simulink model "GPC_model"  (R2022b)
settings: Solver=FixedStepAuto  StartTime=0.0  StopTime=100  FixedStep=0.1  RelTol=1e-3  AbsTol=1e-6
undefined symbols (not defined in the file): DiscIntNeverNeededParam, Ks, Ts
settings Model: ExtModeTrigDuration=12000  ExtModeTrigLevel=0.400000  Creator=jims  LastModifiedBy=artur
settings SolverCC: AutoScaleAbsTol=off  AlgebraicLoopSolver=TrustRegion
settings DataIOCC: ExternalInput=[]  InitialState=[]  MaxDataPoints=5000  SaveFormat=Array  SignalLoggingSaveFormat=ModelDataLogs  SaveOutput=off  SaveTime=off  ReturnWorkspaceOutputs=off  SignalLoggingName=sigsOut
settings OptimizationCC: BooleanDataType=off  ExpressionDepthLimit=2147483647  LifeSpan=inf
settings DebuggingCC: SaveWithParameterizedLinksMsg=none  UnderspecifiedInitializationDetection=Classic  MergeDetectMultiDrivingBlocksExec=none  SignalResolutionControl=TryResolveAllWithWarning  MultiTaskDSMMsg=warning  MultiTaskCondExecSysMsg=none  IntegerOverflowMsg=none  FcnCallInpInsideContextMsg=warning  UnconnectedInputMsg=warning  UnconnectedOutputMsg=warning  UnconnectedLineMsg=warning  AllowSymbolicDim=off  StateNameClashWarn=warning  PregeneratedLibrarySubsystemCodeDiagnostic=none  SFUnexpectedBacktrackingDiag=warning  SFNoUnconditionalDefaultTransitionDiag=warning  SFExecutionAtInitializationDiag=none  SFMachineParentedDataDiag=warning  IntegerSaturationMsg=none  ArithmeticOperatorsInVariantConditions=warning
settings HardwareCC: ProdBitPerLong=64  ProdHWDeviceType=Intel->x86-64 (Linux 64)  TargetBitPerLong=64  TargetBitPerPointer=64  TargetIntDivRoundTo=Zero  TargetEndianess=LittleEndian  TargetWordSize=64  TargetHWDeviceType=Intel->x86-64
settings ModelReferenceCC: EnableRefExpFcnMdlSchedulingChecks=on  PropagateSignalLabelsOutOfModel=off
settings SFSimCC: SimUseLocalCustomCode=off  CustomCodeUndefinedFunction=UseInterfaceOnly
settings RTWCC: Description=Simulink Desktop Real-Time  SystemTargetFile=sldrt.tlc  TemplateMakefile=sldrt.tmf  RTWUseLocalCustomCode=off  RTWCompilerOptimization=on
settings CodeAppCC: MaxIdLength=95  StateflowObjectComments=on
settings SimulinkDesktopRealTimeCC: TargetLibSuffix=_sldrt.a  TargetPreCompLibLocation=C:\Program Files\MATLAB\R2022b\toolbox\sldrt\lib\win64  TargetLangStandard=C89/C90 (ANSI)  SupportVariableSizeSignals=off
settings ConfigComp: CovMetricSettings=dw  CovSaveCumulativeToWorkspaceVar=on  CovSaveSingleToWorkspaceVar=on  CovExternalEMLEnable=off

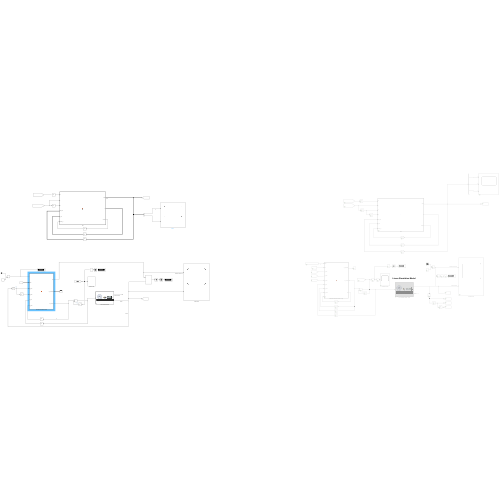
[thumbnail: Simulink's stored preview of the top-level diagram]
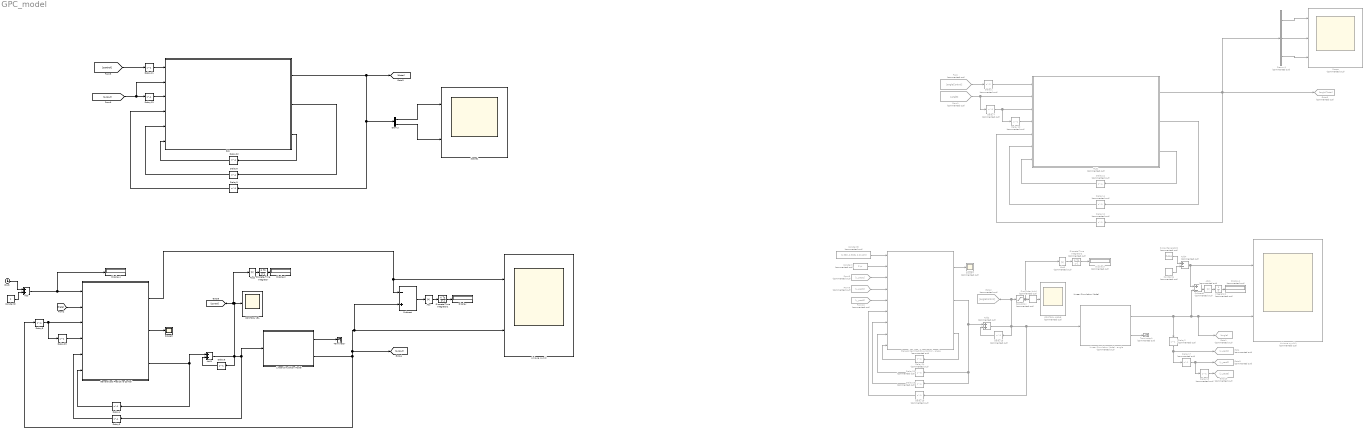
== system GPC_model ==
  note: Linear Simulation Model
  Abs : Abs  SaturateOnIntegerOverflow=off
  Abs1 : Abs  Commented=on  SaturateOnIntegerOverflow=off
  Abs2 : Abs  SaturateOnIntegerOverflow=off
  Abs3 : Abs  Commented=on  SaturateOnIntegerOverflow=off
  Add : Sum
  Add1 : Sum
  Add2 : Sum  Commented=on
  Add4 : Sum  Commented=on  Inputs=+-
  CONTROL ANGLE : Scope  Commented=on
  CONTROL VEL : Scope
  Clock : Clock
  Constant : Constant  Commented=on  Value=2*pi
  Constant2 : Constant
  Constant3 : Constant  Commented=on  Value=[1.988 -0.9884 0.01129]
  Constant4 : Constant  Commented=on  Value=2*3.14
  Delay1 : Delay  Commented=on  InitialCondition=0
  Delay{2,7,10,15..19} (8 alike) : Delay  Commented=on  DelayLength=1  InitialCondition=0
  Delay{3..6,11,13,23} (7 alike) : Delay  DelayLength=1  InitialCondition=0
  Delay12 : Delay  Commented=on  DelayLength=1  InitialCondition=[2.05 -0.95 0.01]
  Delay14 : Delay  Commented=on  DelayLength=1  InitialCondition=eye(3) * 10^6
  Delay20 : Delay  Commented=on  InitialCondition=0
  Delay21 : Delay  Commented=on  DelayLength=1  InitialCondition=10
  Delay22 : Delay  DelayLength=1  InitialCondition=10
  Delay24 : Delay  Commented=on  DelayLength=1  InitialCondition=1
  Delay8 : Delay  DelayLength=1  InitialCondition=eye(2) * 10^6
  Delay9 : Delay  DelayLength=1  InitialCondition=[0.85 21]
  Demux : Demux  Outputs=2
  Demux1 : Demux  Commented=on  Outputs=3
  Discrete-Time Integrator : DiscreteIntegrator  SampleTime=-1  ICPrevOutput=DiscIntNeverNeededParam  ICPrevScaledInput=DiscIntNeverNeededParam
  Discrete-Time Integrator1 : DiscreteIntegrator  SampleTime=-1  ICPrevOutput=DiscIntNeverNeededParam  ICPrevScaledInput=DiscIntNeverNeededParam
  Discrete-Time Integrator2 : DiscreteIntegrator  Commented=on  SampleTime=-1  ICPrevOutput=DiscIntNeverNeededParam  ICPrevScaledInput=DiscIntNeverNeededParam
  Display : Display
  Display1 : Display  Commented=on
  Display2 : Display
  Display3 : Display  Commented=on
  Display4 : Display
  First Order Hold : FirstOrderHold  Commented=on  ErrorTolerance=inf
  From : From  Commented=on  GotoTag=angleControl
  From1 : From  Commented=on  GotoTag=angle
  From10 : From  Commented=on  GotoTag=y_past3
  From8 : From  Commented=on  GotoTag=y_past1
  From9 : From  Commented=on  GotoTag=y_past2
  Generalized Predictive Control : MATLAB Function  TreatAsAtomicUnit=on
  Generalized Predictive Control - angle : MATLAB Function  Commented=on  TreatAsAtomicUnit=on
  Goto : Goto  Commented=on  GotoTag=y_past1
  Goto1 : Goto  Commented=on  GotoTag=angle
  Goto10 : Goto  Commented=on  GotoTag=y_past3
  Goto2 : Goto  Commented=on  GotoTag=angleControl
  Goto5 : Goto  Commented=on  GotoTag=angleTheta
  Goto9 : Goto  Commented=on  GotoTag=y_past2
  Integrator1 : Integrator  Commented=on
  Linear Simulation Model : Subsystem  mask{x0=[0*25*pi/2 0]}
      mask prompts: x0 "Initial conditions [angle vel]"
      mask Display: image(imread('Servo_m.JPG'))
  Linear Simulation Model - angle : Subsystem  Commented=on  mask{x0=[0 0]}
      mask prompts: x0 "Initial conditions [angle vel]"
      mask Display: image(imread('Servo_m.JPG'))
  Liniowe wyniki : Scope  NumInputPorts=2
  Liniowe wyniki1 : Scope  Commented=on  NumInputPorts=2
  Pulse Generator2 : DiscretePulseGenerator  Commented=on  PulseType=Time based  Amplitude=4*pi  Period=4  PulseWidth=50
  RLS : MATLAB Function  TreatAsAtomicUnit=on
  RLS1 : MATLAB Function  Commented=on  TreatAsAtomicUnit=on
  Saturation : Saturate  Commented=on  UpperLimit=1  LowerLimit=-1
  Scope : Scope  Commented=on  NumInputPorts=3
  Scope1 : Scope  NumInputPorts=2
  Scope3 : Scope
  Scope4 : Scope  Commented=on
  Subtract : Sum  Inputs=-+
  Subtract1 : Sum  Commented=on  Inputs=+-
  Terminator : Terminator
  Terminator1 : Terminator  Commented=on
  wires:
  Demux/2 -> Scope1/2  "b1"
  Generalized Predictive Control/3(du_control) -> Add1/1, Delay4/1  "du"
  Delay11/1 -> RLS/1(u1)
  Demux/1 -> Scope1/1  "a1"
  Delay9/1 -> RLS/4(theta_old)
  [control] -> Delay11/1
  Delay4/1 -> Generalized Predictive Control/6(du_past)
  RLS/1(theta) -> Demux/1, Delay9/1, [theta]  "theta"
  Generalized Predictive Control/2(du_predicted) -> Scope3/1
  Delay13/1 -> RLS/3(y1)
  [output] -> Delay13/1, RLS/2(y)
  RLS/2(P) -> Delay8/1
  Delay8/1 -> RLS/5(P_old)
  Delay3/1 -> Generalized Predictive Control/5(u_past)
  [theta] -> Generalized Predictive Control/2(theta)
  Delay6/1 -> Add1/2
  Generalized Predictive Control/1(traj) -> Liniowe wyniki/1, Subtract/1  "Trajektoria referencyjna"
  RLS/3(counter) -> Delay22/1
  Delay22/1 -> RLS/6(counter_p)
  Delay23/1 -> Generalized Predictive Control/4(y_past2)
  Subtract/1 -> Abs/1
  Abs/1 -> Discrete-Time Integrator1/1
  Discrete-Time Integrator1/1 -> Display/1
  RLS1/3(counter) -> Delay21/1
  Delay14/1 -> RLS1/6(P_old)
  From10/1 -> Generalized Predictive Control - angle/5(y_past3)
  Demux1/3 -> Scope/3  "b1"
  Delay21/1 -> RLS1/7(counter_p)
  Generalized Predictive Control - angle/2(du_control) -> Delay16/1, Delay20/1, Add2/1  "du"
  Constant3/1 -> Generalized Predictive Control - angle/1(theta)  "ref"
  Delay2/1 -> Delay17/1, Goto/1
  From8/1 -> Generalized Predictive Control - angle/3(y_past1)
  Constant4/1 -> Add4/2
  Generalized Predictive Control - angle/1(du_predicted) -> Scope4/1
  Pulse Generator2/1 -> Add4/1
  Demux1/1 -> Scope/1  "a1"
  Delay7/1 -> Delay10/1, RLS1/3(y1)
  Delay18/1 -> Goto10/1
  From9/1 -> Generalized Predictive Control - angle/4(y_past2)
  Add2/1 -> Saturation/1, Goto2/1, Delay15/1, Linear Simulation Model - angle/1(Control), Delay19/1  "S"
  RLS1/2(P) -> Delay14/1
  Constant/1 -> Generalized Predictive Control - angle/2(ref)
  Generalized Predictive Control - angle/3(cnt) -> Delay24/1
  Delay15/1 -> Add2/2
  RLS1/1(theta) -> Delay12/1, Goto5/1, Demux1/1
  Delay20/1 -> Generalized Predictive Control - angle/8(du_past2)
  From1/1 -> Delay7/1, RLS1/2(y)
  Delay1/1 -> RLS1/1(u2)
  Linear Simulation Model - angle/2(Velocity) -> Terminator1/1  "Velocity"
  Delay12/1 -> RLS1/5(theta_old)
  From/1 -> Delay1/1
  Add4/1 -> Liniowe wyniki1/1, Subtract1/1  "Trajektoria referencyjna"
  Delay24/1 -> Generalized Predictive Control - angle/9(cntp)
  Linear Simulation Model - angle/1(Angle) -> Delay2/1, Liniowe wyniki1/2, Goto1/1, Subtract1/2  "Położenie kątowe"
  Delay16/1 -> Generalized Predictive Control - angle/7(du_past1)
  Demux1/2 -> Scope/2  "a2"
  Delay10/1 -> RLS1/4(y2)
  Delay19/1 -> Generalized Predictive Control - angle/6(u_past)
  Delay17/1 -> Delay18/1, Goto9/1
  Subtract1/1 -> Abs1/1
  Abs1/1 -> Integrator1/1
  Integrator1/1 -> Display1/1
  First Order Hold/1 -> CONTROL ANGLE/1
  Saturation/1 -> Abs3/1, First Order Hold/1
  Linear Simulation Model/2(Velocity) -> Delay5/1, Subtract/2, Liniowe wyniki/2, [output]  "Velocity"
  Discrete-Time Integrator/1 -> Display2/1
  Abs2/1 -> Discrete-Time Integrator/1
  Abs3/1 -> Discrete-Time Integrator2/1
  Discrete-Time Integrator2/1 -> Display3/1
  Add1/1 -> Linear Simulation Model/1(Control), Delay3/1, Abs2/1, [control], CONTROL VEL/1, Delay6/1
  Add/1 -> Display4/1, Generalized Predictive Control/1(t)
  Clock/1 -> Add/1
  Constant2/1 -> Add/2
  Delay5/1 -> Delay23/1, Generalized Predictive Control/3(y_past1)
  Linear Simulation Model/1(Angle) -> Terminator/1  "Położenie kątowe"

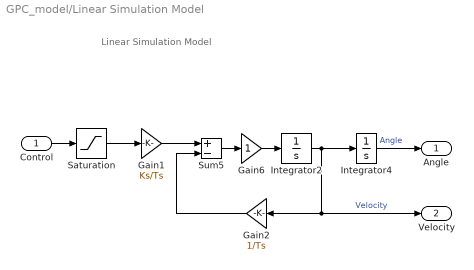
== system GPC_model/Linear Simulation Model ==
  note: Linear Simulation Model
  Control : Inport
  Gain1 : Gain  Gain=Ks/Ts  SaturateOnIntegerOverflow=on  OutDataTypeStr=Inherit: Same as input  ParamDataTypeStr=Inherit: Same as input
  Gain2 : Gain  Gain=1/Ts  SaturateOnIntegerOverflow=on  OutDataTypeStr=Inherit: Same as input  ParamDataTypeStr=Inherit: Same as input
  Gain6 : Gain  SaturateOnIntegerOverflow=on  OutDataTypeStr=Inherit: Same as input  ParamDataTypeStr=Inherit: Same as input
  Integrator2 : Integrator  InitialCondition=x0(2)
  Integrator4 : Integrator  InitialCondition=x0(1)
  Saturation : Saturate  UpperLimit=1  LowerLimit=-1
  Sum5 : Sum  Inputs=+-  InputSameDT=on  SaturateOnIntegerOverflow=on  OutDataTypeStr=Inherit: Same as first input
  Angle : Outport  InitialOutput=0  VectorParamsAs1DForOutWhenUnconnected=off
  Velocity : Outport  Port=2  InitialOutput=0  VectorParamsAs1DForOutWhenUnconnected=off
  wires:
  Sum5/1 -> Gain6/1
  Gain2/1 -> Sum5/2
  Integrator2/1 -> Integrator4/1, Velocity/1, Gain2/1  "Velocity"
  Integrator4/1 -> Angle/1  "Angle"
  Gain6/1 -> Integrator2/1
  Control/1 -> Saturation/1
  Gain1/1 -> Sum5/1
  Saturation/1 -> Gain1/1

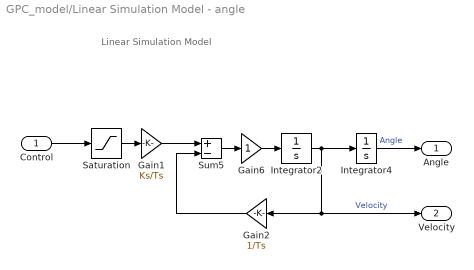
== system GPC_model/Linear Simulation Model - angle ==
  note: Linear Simulation Model
  Control : Inport
  Gain1 : Gain  Gain=Ks/Ts  SaturateOnIntegerOverflow=on  OutDataTypeStr=Inherit: Same as input  ParamDataTypeStr=Inherit: Same as input
  Gain2 : Gain  Gain=1/Ts  SaturateOnIntegerOverflow=on  OutDataTypeStr=Inherit: Same as input  ParamDataTypeStr=Inherit: Same as input
  Gain6 : Gain  SaturateOnIntegerOverflow=on  OutDataTypeStr=Inherit: Same as input  ParamDataTypeStr=Inherit: Same as input
  Integrator2 : Integrator  InitialCondition=x0(2)
  Integrator4 : Integrator  InitialCondition=x0(1)
  Saturation : Saturate  UpperLimit=1  LowerLimit=-1
  Sum5 : Sum  Inputs=+-  InputSameDT=on  SaturateOnIntegerOverflow=on  OutDataTypeStr=Inherit: Same as first input
  Angle : Outport  InitialOutput=0  VectorParamsAs1DForOutWhenUnconnected=off
  Velocity : Outport  Port=2  InitialOutput=0  VectorParamsAs1DForOutWhenUnconnected=off
  wires:
  Sum5/1 -> Gain6/1
  Gain2/1 -> Sum5/2
  Integrator2/1 -> Integrator4/1, Velocity/1, Gain2/1  "Velocity"
  Integrator4/1 -> Angle/1  "Angle"
  Gain6/1 -> Integrator2/1
  Control/1 -> Saturation/1
  Saturation/1 -> Gain1/1
  Gain1/1 -> Sum5/1

== matlab function GPC_model/Generalized Predictive Control ==
  data: t input; traj output; du_predicted output; theta input; y_past1 input; y_past2 input; u_past input; du_past input; du_control output
function [traj,du_predicted, du_control] = fcn(t,theta,y_past1,y_past2,u_past,du_past)

%Współczynniki modelu z algorytmu RLS
a1 = -theta(1);
b1 = theta(2);

%Przeszłe wyjścia
y_past = [y_past1;y_past2];
    
%Parametry
ny = 60; %HORYZONT PREDYKCJI
nu = 24; %HORYZONT STEROWANIA
lambda = 0.01;
    
%Czy wykorzystać T-filtr?
filtrowanie = false;
    
%Ustawienie ograniczeń dla optymalizatora 
%true - ograniczenia na y, false - bez ograniczeń na y
ograniczenie_wyjscia = false;

du_max = 0.1;
du_min = -0.1;
u_max = 1;
u_min = -1;
y_max = 52;
y_min = -52;

%Trajektoria referencyjna
Ts = 0.1; sim_time = 100; ref = 194;

traj_ub = ref*ones(1/Ts*sim_time/2,1);

traj_lb = -ref*ones(1/Ts*sim_time/2,1);

trajektoria = [traj_ub;traj_lb;traj_lb;-ref*ones(ny,1)];

ref = trajektoria(fix(t/Ts):ny+fix(t/Ts)-1, 1);

traj = ref(1);

%%%

    %Wyznaczenie wielomianów a i b
    a = [1 a1];
    b = [0 b1];
    A = conv(a,[1 -1]);
    
    %Wyznaczenie macierzy predykcji
    [Ca,Ha] = predmat(A,ny);
    [Cb,Hb] = predmat(b,ny);
    
    Cai = inv(Ca);
    
    H = Cai*Cb;
    P = Cai*Hb;
    Q = Cai*(-Ha);

%%%%%%%%%%%%%%%%%%%%%%%%%%%%%%%%%%%%%%%%%%%%%%%%%%%%%%%%%%%%%%%%%%%%%%%%%%%

if filtrowanie == true
    Tfilt = [1 -0.2];
    
    [Ct,Ht] = predmat(Tfilt,ny);
    Pt = Ct * P - H * Ht;
    Qt = Ct * Q + Ht;
    
    P = Pt;
    Q = Qt;
end

%%%%%%%%%%%%%%%%%%%%%%%%%%%%%%%%%%%%%%%%%%%%%%%%%%%%%%%%%%%%%%%%%%%%%%%%%%%

    Hu = H(:,1:nu); %horyzont sterowania

%Prawo sterowania dla algorytmu z ograniczeniami
    S = Hu'*Hu + eye(nu)*lambda;
    S = (S + S')/2;
    f = Hu'*Q * y_past + Hu'*P * du_past - Hu' * ref;

    if ograniczenie_wyjscia == true
        %OGRANICZENIA Z Y
        [C,dd,du,ddu,dy] = mpc_ograniczenia(du_max, du_min,u_max,u_min,y_max,y_min,nu,Hu,P,Q,1,2);
        dt = dd + du * u_past + ddu * du_past + dy*y_past;
    else
        %OGRANICZENIA BEZ Y
        [C, dd,du] = mpc_ograniczenia_bez_y(du_max,du_min,u_max,u_min,nu);
        dt = dd + du * u_past;
    end


    opts = optimoptions('quadprog','Algorithm','active-set');

    x0 = 0*eye(nu,1);

    du_predicted = quadprog(S,f,C,dt,[],[],[],[],x0,opts);

    du_control = du_predicted(1);


%Prawo sterowania dla algorytmu bez ograniczeń
% Pr = ( inv(Hu'*Hu+lambda*eye(nu)) ) * Hu';
% Nk = Pr*Q;
% Dk = Pr*P;
% 
% du_predicted = Pr * ref - Dk * du_past - Nk*y_past;
% du_control = du_predicted(1);

== matlab function GPC_model/RLS1 ==
  data: u2 input; y input; y1 input; y2 input; theta output; theta_old input; P_old input; P output; counter_p input; counter output
function [theta,P,counter]= fcn(u2,y,y1,y2,theta_old,P_old,counter_p)

counter = counter_p;

lambda = 0.985;

phi = [y1;y2;u2];

if counter_p == 10

K = P_old * phi/(lambda + phi'*P_old*phi);

P = ((eye(3) - K * phi') * P_old) * lambda^-1;

theta = theta_old + K * (y - phi'*theta_old);

counter = 1;
else

theta = theta_old;
P = P_old;
counter = counter + 1;
end

== matlab function GPC_model/Generalized Predictive Control - angle ==
  data: du_predicted output; theta input; ref input; y_past1 input; y_past2 input; y_past3 input; u_past input; du_past1 input; du_control output; du_past2 input; cnt output; cntp input
function [du_predicted, du_control,cnt] = fcn(theta,ref,y_past1,y_past2,y_past3,u_past,du_past1,du_past2,cntp)

cnt = cntp;

%Współczynniki modelu z algorytmu RLS
a1 = -theta(1);
a2 = -theta(2);
b1 = theta(3);

%Parametry
ny = 20; %HORYZONT PREDYKCJI
nu = 12; %HORYZONT STEROWANIA
lambda = 0.45;

%Przeszłe wyjścia
y_past = [y_past1;y_past2;y_past3];
du_past = [du_past1;du_past2];

%Trajektoria referencyjna, stała

%Trajektoria referencyjna, stała
Ts = 0.01; %PRÓBKOWANIE SYMULACJI
sim_time = 4; %CZAS SYMULACJI

traj_ub = ref*ones(1/Ts*sim_time/2,1);

traj_lb = -ref*ones(1/Ts*sim_time/2,1);

%%% trajektoria referencyjna
trajektoria = [traj_ub;traj_lb;traj_ub;-ref*ones(ny,1)];

ref = trajektoria(cnt:ny+cnt-1, 1);

cnt = cntp + 1;

%%%

%Czy wykorzystać T-filtr?
filtrowanie = false;

%Ograniczenia
%true - ograniczenia na y, false - bez ograniczeń na y
ograniczenie_wyjscia = true;

du_max = 1;
du_min = -1;
u_max = 1;
u_min = -1;
y_max = 6.6;
y_min = -6.6;

%Wyznaczenie wielomianów a i b
a = [1 a1 a2];
b = [0 0 b1];
A = conv(a,[1 -1]);

%Wyznaczenie macierzy predykcji
[Ca,Ha] = predmat(A,ny);
[Cb,Hb] = predmat(b,ny);

Cai = inv(Ca);

H = Cai*Cb;
P = Cai*Hb;
Q = Cai*(-Ha);

%%%%%%%%%%%%%%%%%%%%%%%%%%%%%%%%%%%%%%%%%%%%%%%%%%%%%%%%%%%%%%%%%%%%%%%%%%%

if filtrowanie == true
    Tfilt = [1 -0.05];
    
    [Ct,Ht] = predmat(Tfilt,ny);
    Pfilt = Ct * P - H * Ht;
    Qfilt = Ct * Q + Ht;
    
    P = Pfilt;
    Q = Qfilt;
end

%%%%%%%%%%%%%%%%%%%%%%%%%%%%%%%%%%%%%%%%%%%%%%%%%%%%%%%%%%%%%%%%%%%%%%%%%%%

Hu = H(:,1:nu); %horyzont sterowania

%Ustawienie ograniczeń dla optymalizatora 

%Prawo sterowania dla algorytmu z ograniczeniami
S = Hu'*Hu + eye(nu)*lambda;
S = (S + S')/2;
f = Hu'*Q * y_past + Hu'*P * du_past - Hu' * ref;

    if ograniczenie_wyjscia == true
        %OGRANICZENIA Z Y
        [C,dd,du,ddu,dy] = mpc_ograniczenia(du_max, du_min,u_max,u_min,y_max,y_min,nu,Hu,P,Q,2,3);
        dt = dd + du * u_past + ddu * du_past + dy*y_past;
    else
        %OGRANICZENIA BEZ Y
        [C, dd,du] = mpc_ograniczenia_bez_y(du_max,du_min,u_max,u_min,nu);
        dt = dd + du * u_past;
    end


opts = optimoptions('quadprog','Algorithm','active-set');

x0 = 0*eye(nu,1);

du_predicted = quadprog(S,f,C,dt,[],[],[],[],x0,opts);

du_control = du_predicted(1);

%Prawo sterowania dla algorytmu bez ograniczeń
% Pr = ( inv(Hu'*Hu+lambda*eye(nu)) ) * Hu';
% Nk = Pr*Q;
% Dk = Pr*P;
% 
% du_predicted = Pr * ref - Dk * du_past - Nk*y_past;
% du_control = du_predicted(1);

== matlab function GPC_model/RLS ==
  data: u1 input; y input; y1 input; theta output; theta_old input; P_old input; P output; counter_p input; counter output
function [theta,P,counter]= fcn(u1,y,y1,theta_old,P_old,counter_p)

counter = counter_p;

if counter_p == 10

lambda = 0.985;
phi = [y1;u1];

K = P_old * phi/(lambda + phi'*P_old*phi);

P = ((eye(2) - K * phi') * P_old) * lambda^-1;

theta = theta_old + K * (y - phi'*theta_old);

counter = 1;
else
    theta = theta_old;
    P = P_old;
    counter = counter + 1;
end
